simulink model "Filtri_Statici"  (R2022b)
settings: Solver=VariableStepAuto  StartTime=0.0  StopTime=time_max  FixedStep=1e-6  RelTol=1e-4
values from neighbouring files (symbols this model uses):
  bias_accel = [bias_a_x; bias_a_y; bias_a_z]    [Main_Articolo.m]
  bias_csi = [bias_csi_x; bias_csi_y; bias_csi_z]    [Main_Articolo.m]
  bias_gyro = [bias_gyro_x; bias_gyro_y; bias_gyro_z]    [Main_Articolo.m]    (also in Plot_Filtri_Din.m = out.bias_gyro.Data)
  bias_magn = [bias_magn_x; bias_magn_y; bias_magn_z]    [Main_Articolo.m]
  csi_i = [0; csi_y_i; 0]    [Main_Articolo.m]
  dev_std_a_x = 0.0248    [Main_Articolo.m]
  dev_std_a_y = 0.0248    [Main_Articolo.m]
  dev_std_a_z = 0.0203    [Main_Articolo.m]
  dev_std_csi_x = 0.01    [Main_Articolo.m]
  dev_std_csi_y = 0.007    [Main_Articolo.m]
  dev_std_csi_z = 0.005    [Main_Articolo.m]
  dev_std_gyro_x = 2.653*10^(-3)    (= 0.002653)    [Main_Articolo.m]
  dev_std_gyro_y = 2.653*10^(-3)    (= 0.002653)    [Main_Articolo.m]
  dev_std_gyro_z = 3.159*10^(-3)    (= 0.003159)    [Main_Articolo.m]
  dev_std_magn_x = 0.01    [Main_Articolo.m]
  dev_std_magn_y = 0.015    [Main_Articolo.m]
  dev_std_magn_z = 0.0175    [Main_Articolo.m]
  dt = 0.01    [Main_Articolo.m]
  flag = 1    [Main_Articolo.m]
  g = 9.81    [Main_Articolo.m]
  index = 0    [Main_Articolo.m]
  k_accel = 1/3    (= 0.333333333333)    [Main_Articolo.m]
  k_csi = 1/3    (= 0.333333333333)    [Main_Articolo.m]
  k_magn = 1/3    (= 0.333333333333)    [Main_Articolo.m]
  m_I = [m_i_x; 0; m_i_z]    [Main_Articolo.m]
  Omega11 = 0.075    [Main_Articolo.m]
  Omega12 = 0.045    [Main_Articolo.m]
  Omega13 = 0.02    [Main_Articolo.m]
  Omega21 = 0.085    [Main_Articolo.m]
  Omega22 = -0.03    [Main_Articolo.m]
  Omega23 = 0.015    [Main_Articolo.m]
  Omega31 = 0.1    [Main_Articolo.m]
  Omega32 = 0.036    [Main_Articolo.m]
  Omega33 = -0.025    [Main_Articolo.m]
  Phi1 = 40*pi/180    (= 0.698131700798)    [Main_Articolo.m]
  Phi2 = 20*pi/180    (= 0.349065850399)    [Main_Articolo.m]
  Phi3 = 2*pi/180    (= 0.0349065850399)    [Main_Articolo.m]
  phi_0 = 15*pi/180    (= 0.261799387799)    [Main_Articolo.m]
  pos_0 = [x_0; y_0; z_0]    [Main_Articolo.m]
  Psi1 = 160*pi/180    (= 2.79252680319)    [Main_Articolo.m]
  Psi2 = 35*pi/180    (= 0.610865238198)    [Main_Articolo.m]
  Psi3 = 5*pi/180    (= 0.0872664625997)    [Main_Articolo.m]
  psi_0 = pi/4    (= 0.785398163397)    [Main_Articolo.m]
  rumori_bias = 1    [Main_Articolo.m]
  Theta1 = 50*pi/180    (= 0.872664625997)    [Main_Articolo.m]
  Theta2 = 12*pi/180    (= 0.209439510239)    [Main_Articolo.m]
  Theta3 = 3*pi/180    (= 0.0523598775598)    [Main_Articolo.m]
  theta_0 = 10*pi/180    (= 0.174532925199)    [Main_Articolo.m]
  Ttriad = 1/30    (= 0.0333333333333)    [Main_Articolo.m]
  vel_0 = [dx_0; dy_0; dz_0]    [Main_Articolo.m]
  w_11 = 2*pi/30    (= 0.209439510239)    [Main_Articolo.m]
  w_12 = 2*pi/12    (= 0.523598775598)    [Main_Articolo.m]
  w_13 = 2*pi/4    (= 1.57079632679)    [Main_Articolo.m]
  w_21 = 2*pi/25    (= 0.251327412287)    [Main_Articolo.m]
  w_22 = 2*pi/18    (= 0.349065850399)    [Main_Articolo.m]
  w_23 = 2*pi/3    (= 2.09439510239)    [Main_Articolo.m]
  w_31 = 2*pi/20    (= 0.314159265359)    [Main_Articolo.m]
  w_32 = 2*pi/10    (= 0.628318530718)    [Main_Articolo.m]
  w_33 = 2*pi/2    (= 3.14159265359)    [Main_Articolo.m]
  w_phi1 = 2*pi/27    (= 0.232710566933)    [Main_Articolo.m]
  w_phi2 = 2*pi/18    (= 0.349065850399)    [Main_Articolo.m]
  w_phi3 = 2*pi/3    (= 2.09439510239)    [Main_Articolo.m]
  w_psi1 = 2*pi/30    (= 0.209439510239)    [Main_Articolo.m]
  w_psi2 = 2*pi/15    (= 0.418879020479)    [Main_Articolo.m]
  w_psi3 = 2*pi/4    (= 1.57079632679)    [Main_Articolo.m]
  w_theta1 = 2*pi/23    (= 0.273181969877)    [Main_Articolo.m]
  w_theta2 = 2*pi/12    (= 0.523598775598)    [Main_Articolo.m]
  w_theta3 = 2*pi/3.5    (= 1.79519580205)    [Main_Articolo.m]
settings Model: Creator=paoga  LastModifiedBy=paoga

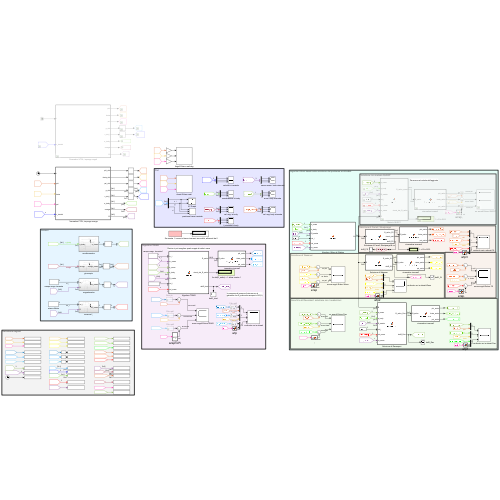
[thumbnail: Simulink's stored preview of the top-level diagram]
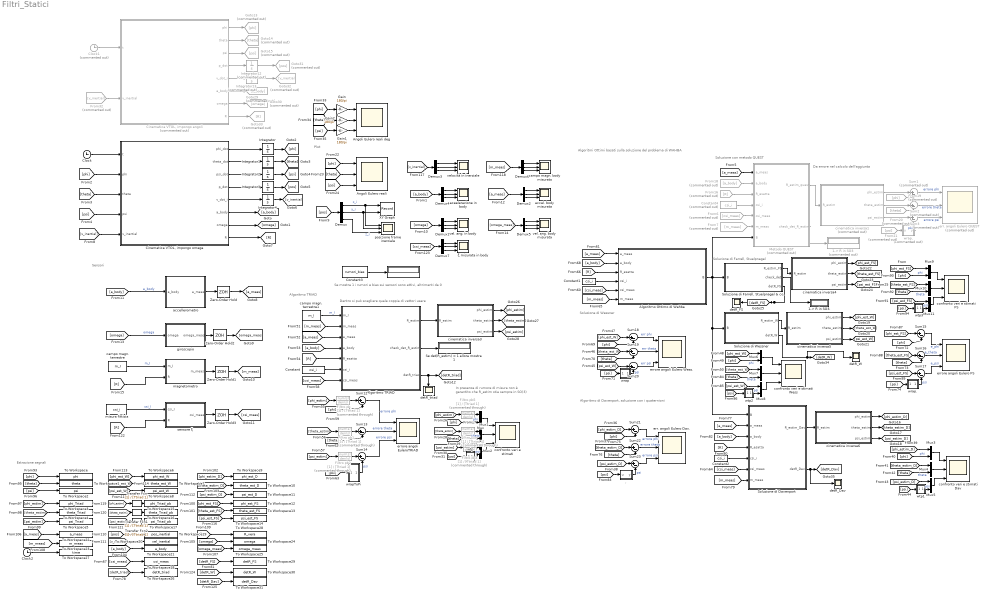
== system Filtri_Statici ==
  note: Da errore nel calcolo dell'aggiunta
  note: Algoritmi Ottimi basati sulla soluzione del problema di WAHBA
  note: Soluzione con metodo QUEST
  note: Algoritmo di Davenport, soluzione con i quaternioni
  note: Plot
  note: Sensori
  note: Dentro si può scegliere quale coppia di vettori usare
  note: In presenza di rumore di misura non è
      | garantito che R_estim stia sempre in SO(3)
  note: Algoritmo TRIAD
  note: Soluzione di Wessner
  note: Soluzione di Farrell, Stuelpnagel
  note: Se mostra 1 i rumori e bias sui sensori sono attivi, altrimenti da 0
  note: Estrazione segnali
  , : MATLAB Function  TreatAsAtomicUnit=on
  . : Display
  1-> R in SO3 : Display  Commented=on
  1-> R in SO3. : Display
  Algoritmo Ottimo di Wahba : MATLAB Function  TreatAsAtomicUnit=on
  Algoritmo TRIAD : MATLAB Function  TreatAsAtomicUnit=on
  Angoli Eulero reali : Scope  NumInputPorts=3
  Angoli Eulero reali deg : Scope  NumInputPorts=3
  "Cinematica VTOL, impongo angoli" : MATLAB Function  Commented=on  TreatAsAtomicUnit=on
  "Cinematica VTOL, impongo omega" : MATLAB Function  TreatAsAtomicUnit=on
  Clock : Clock
  Clock1 : Clock  Commented=on
  Clock2 : Clock
  Constant : Constant  Value=csi_i
  Constant1 : Constant  Value=csi_i
  Constant2 : Constant  Value=csi_i
  Constant3 : Constant  Value=rumori_bias
  Constant4 : Constant  Commented=on  Value=csi_i
  Demux{,1..7} (8 alike) : Demux  Outputs=3
  Filtro pb{,1..5} (6 alike) : TransferFcn  Commented=through  Denominator=[Ttriad 1]
  From16 : From  Commented=on  GotoTag=R
  From18 : From  Commented=on  GotoTag=a_body
  From19 : From  Commented=on  GotoTag=phi
  From20 : From  Commented=on  GotoTag=theta
  From21 : From  Commented=on  GotoTag=psi
  From32 : From  Commented=on  GotoTag=v_inertial
  From6 : From  Commented=on  GotoTag=csi_meas
  From7 : From  Commented=on  GotoTag=m_meas
  Gain : Gain  Gain=180/pi
  Gain1 : Gain  Gain=180/pi
  Gain2 : Gain  Gain=180/pi
  Goto13 : Goto  Commented=on  GotoTag=phi
  Goto14 : Goto  Commented=on  GotoTag=theta
  Goto15 : Goto  Commented=on  GotoTag=psi
  Goto29 : Goto  Commented=on  GotoTag=a_body
  Goto30 : Goto  Commented=on  GotoTag=omega
  Goto31 : Goto  Commented=on  GotoTag=pos
  Goto32 : Goto  Commented=on  GotoTag=v_inertial
  Goto33 : Goto  Commented=on  GotoTag=R
  Integrator : Integrator  InitialCondition=phi_0
  Integrator1 : Integrator  InitialCondition=theta_0
  Integrator12 : Integrator  Commented=on  InitialCondition=pos_0
  Integrator13 : Integrator  Commented=on  InitialCondition=vel_0
  Integrator2 : Integrator  InitialCondition=psi_0
  Integrator3 : Integrator  InitialCondition=pos_0
  Integrator4 : Integrator  InitialCondition=vel_0
  Metodo QUEST : MATLAB Function  Commented=on  TreatAsAtomicUnit=on
  Mux{,1..11} (12 alike) : Mux  Inputs=2
  Se det(R_estim) = 1 allora mostra 1 : Display
  Soluzione di Davenport : MATLAB Function  TreatAsAtomicUnit=on
  "Soluzione di Farrell, Stuelpnagel & co." : MATLAB Function  TreatAsAtomicUnit=on
  Soluzione di Wessner : MATLAB Function  TreatAsAtomicUnit=on
  Sum1 : Sum  Commented=on  Inputs=|+-
  Sum{12..23} (12 alike) : Sum  Inputs=|+-
  Sum2 : Sum  Commented=on  Inputs=|+-
  Sum3 : Sum  Commented=on  Inputs=|+-
  To Workspace : ToWorkspace  VariableName=phi  SaveFormat=Timeseries  SampleTime=-1
  To Workspace1 : ToWorkspace  VariableName=theta  SaveFormat=Timeseries  SampleTime=-1
  To Workspace10 : ToWorkspace  VariableName=theta_est_D  SaveFormat=Timeseries  SampleTime=-1
  To Workspace11 : ToWorkspace  VariableName=psi_est_D  SaveFormat=Timeseries  SampleTime=-1
  To Workspace12 : ToWorkspace  VariableName=phi_est_FS  SaveFormat=Timeseries  SampleTime=-1
  To Workspace13 : ToWorkspace  VariableName=theta_est_FS  SaveFormat=Timeseries  SampleTime=-1
  To Workspace14 : ToWorkspace  VariableName=psi_est_FS  SaveFormat=Timeseries  SampleTime=-1
  To Workspace15 : ToWorkspace  VariableName=phi_Triad_pb  SaveFormat=Timeseries  SampleTime=-1
  To Workspace16 : ToWorkspace  VariableName=theta_Triad_pb  SaveFormat=Timeseries  SampleTime=-1
  To Workspace17 : ToWorkspace  VariableName=psi_Triad_pb  SaveFormat=Timeseries  SampleTime=-1
  To Workspace18 : ToWorkspace  VariableName=csi_meas  SaveFormat=Timeseries  SampleTime=-1
  To Workspace19 : ToWorkspace  VariableName=pos_inertial  SaveFormat=Timeseries  SampleTime=-1
  To Workspace2 : ToWorkspace  VariableName=psi  SaveFormat=Timeseries  SampleTime=-1
  To Workspace20 : ToWorkspace  VariableName=vel_inertial  SaveFormat=Timeseries  SampleTime=-1
  To Workspace21 : ToWorkspace  VariableName=a_body  SaveFormat=Timeseries  SampleTime=-1
  To Workspace22 : ToWorkspace  VariableName=a_meas  SaveFormat=Timeseries  SampleTime=-1
  To Workspace23 : ToWorkspace  VariableName=m_meas  SaveFormat=Timeseries  SampleTime=-1
  To Workspace24 : ToWorkspace  VariableName=omega  SaveFormat=Timeseries  SampleTime=-1
  To Workspace25 : ToWorkspace  VariableName=omega_meas  SaveFormat=Timeseries  SampleTime=-1
  To Workspace26 : ToWorkspace  VariableName=detR_triad  SaveFormat=Timeseries  SampleTime=-1
  To Workspace27 : ToWorkspace  VariableName=time  SampleTime=-1
  To Workspace28 : ToWorkspace  VariableName=R_vera  SampleTime=-1
  To Workspace29 : ToWorkspace  VariableName=detR_FS  SaveFormat=Timeseries  SampleTime=-1
  To Workspace3 : ToWorkspace  VariableName=phi_Triad  SaveFormat=Timeseries  SampleTime=-1
  To Workspace30 : ToWorkspace  VariableName=detR_W  SaveFormat=Timeseries  SampleTime=-1
  To Workspace31 : ToWorkspace  VariableName=detR_Dav  SaveFormat=Timeseries  SampleTime=-1
  To Workspace4 : ToWorkspace  VariableName=theta_Triad  SaveFormat=Timeseries  SampleTime=-1
  To Workspace5 : ToWorkspace  VariableName=psi_Triad  SaveFormat=Timeseries  SampleTime=-1
  To Workspace6 : ToWorkspace  VariableName=phi_est_W  SaveFormat=Timeseries  SampleTime=-1
  To Workspace7 : ToWorkspace  VariableName=theta_est_W  SaveFormat=Timeseries  SampleTime=-1
  To Workspace8 : ToWorkspace  VariableName=psi_est_W  SaveFormat=Timeseries  SampleTime=-1
  To Workspace9 : ToWorkspace  VariableName=phi_est_D  SaveFormat=Timeseries  SampleTime=-1
  Transfer Fcn : TransferFcn  Denominator=[Ttriad 1]
  Transfer Fcn1 : TransferFcn  Denominator=[Ttriad 1]
  Transfer Fcn2 : TransferFcn  Denominator=[Ttriad 1]
  XY Graph : Record  FileSettingsInternal="{\"entries\":[{\"content\":{\"excelSettings\":{\"content\":{},\"type\":\"Streamout.ExcelSettings\"}},\"type\":\"Streamout.FileSettingStorage\",\"uuid\":\"477e70b2-955e-4b5a-84c2-a5f2bc9940fe\"}],\"packageUris\":[\"http://schema.mathworks.com/mf0/streamout_blocks/R2020a\"],\"version\":\"1.0\"}"  Layout=[1 1]  SignalsInternal="{\"entries\":[{\"content\":{\"signals\":[{\"content\":{\"blockPath\":[\"Filtri_Statici/XY Graph\"],\"channel\":[],\"dimensions\":[1,1],\"domain\":\"Filtri_Statici/XY Graph\",\"lineColor\":\"#a2142f\",\"plots\":[1],\"port\":1,\"sid\":[\"\"],\"signalID\":3592,\"signalName\":\"x_i\"},\"type\":\"RecordBlkView.Signal\",\"uuid\":\"d6606014-7fdd-4c5b-a990-e5a37003c0d6\"},{\"content\":{\"blockPath\":[\"Filtri_Statici/XY Graph\"],\"channel\":[],\"dimensions\":[1,1],\"domain\":\"Filtri_Statici/XY Graph\",\"lineColor\":\"#139fff\",\"plots\":[1],\"port\":2,\"sid\":[\"\"],\"signalID\":3596,\"signalName\":\"y_i\"},\"type\":\"RecordBlkView.Signal\",\"uuid\":\"6f7c022e-9ea7-4631-a991-0923b55dc0a6\"}]},\"type\":\"RecordBlkView.InputSignals\",\"uuid\":\"fece2fe3-a12d-44ca-a4d1-88af198f26aa\"}],\"packageUris\":[\"http://schema.mathworks.com/mf0/streamout_blocks/R2020a\"],\"version\":\"1.0\"}"  VisualizationBindings="{\"xyplotplugin\":{\"info\":[{\"series\":[{\"bindingParametersList\":[{\"parameter\":\"X-Axis\",\"signalID\":3592,\"signalName\":\"x_i\"},{\"parameter\":\"Y-Axis\",\"signalID\":3596,\"signalName\":\"y_i\"}],\"seriesID\":16300}],\"subplotID\":1}]}}"  CompatibilityTag=XY
  Zero-Order Hold{,1..3} (4 alike) : ZeroOrderHold  SampleTime=dt
  accel. body misurata : Scope  NumInputPorts=3
  accellerometro : Subsystem
  aceelerazione in body : Scope  NumInputPorts=3
  campo magn. body misurato : Scope  NumInputPorts=3
  campo magn. terrestre : Constant  Value=m_I
  campo magn. terrestre1 : Constant  Value=m_I
  cinematica inversa1 : MATLAB Function  Commented=on  TreatAsAtomicUnit=on
  cinematica inversa3 : MATLAB Function  TreatAsAtomicUnit=on
  cinematica inversa4 : MATLAB Function  TreatAsAtomicUnit=on
  cinematica inversa5 : MATLAB Function  TreatAsAtomicUnit=on
  cinematica inversa6 : MATLAB Function  TreatAsAtomicUnit=on
  confronto veri e stimati : Scope  NumInputPorts=3
  confronto veri e stimati Dav : Scope  NumInputPorts=3
  confronto veri e stimati FS : Scope  NumInputPorts=3
  confronto veri e stimati Wess : Scope  NumInputPorts=3
  detR_Dav : Scope
  detR_FS : Scope
  detR_W : Scope
  detR_triad : Scope
  err. angoli Eulero Dav. : Scope  NumInputPorts=3
  err. angoli Eulero QUEST : Scope  Commented=on  NumInputPorts=3
  errore angoli Eulero FS : Scope  NumInputPorts=3
  errore angoli Eulero Wess. : Scope  NumInputPorts=3
  errore angoli EuleroTRIAD : Scope  NumInputPorts=3
  giroscopio : Subsystem
  magnetometro : Subsystem
  misura fittizia : Constant  Value=csi_i
  posizione frame inerziale : Scope  NumInputPorts=3
  "sensore ξ " : Subsystem
  vel. ang. body misurata : Scope  NumInputPorts=3
  vel. ang. in body : Scope  NumInputPorts=3
  velocità in inerziale : Scope  NumInputPorts=3
  wrap : MATLAB Function  TreatAsAtomicUnit=on
  wrap, : MATLAB Function  Commented=on  TreatAsAtomicUnit=on
  wrap. : MATLAB Function  TreatAsAtomicUnit=on
  wrapToPi : MATLAB Function  TreatAsAtomicUnit=on
  wtp : MATLAB Function  TreatAsAtomicUnit=on
  wtp1 : MATLAB Function  TreatAsAtomicUnit=on
  wtp2 : MATLAB Function  TreatAsAtomicUnit=on
  wtp3 : MATLAB Function  TreatAsAtomicUnit=on
  ξ misurata in body : Scope  NumInputPorts=3
  wires:
  Demux1/3 -> vel. ang. in body/3
  "Cinematica VTOL, impongo omega"/6(a_body) -> [a_body]
  Integrator/1 -> [phi]
  [psi] -> "Cinematica VTOL, impongo omega"/4(psi)
  [omega] -> Demux1/1
  Clock/1 -> "Cinematica VTOL, impongo omega"/1(t)
  Demux5/3 -> vel. ang. body misurata/3
  Integrator4/1 -> [v_inertial]
  Demux4/1 -> aceelerazione in body/1
  Integrator2/1 -> [psi]
  Constant3/1 -> ./1
  [a_meas] -> Demux2/1
  [omega_meas] -> Demux5/1
  [a_body] -> Demux4/1
  Demux4/2 -> aceelerazione in body/2
  "Cinematica VTOL, impongo omega"/7(omega) -> [omega]
  [pos] -> Demux/1
  Demux/1 -> posizione frame inerziale/1, XY Graph/1  "x_i"
  [phi] -> "Cinematica VTOL, impongo omega"/2(phi)
  Integrator3/1 -> [pos]
  Demux2/1 -> accel. body misurata/1
  Demux2/2 -> accel. body misurata/2
  [v_inertial] -> "Cinematica VTOL, impongo omega"/5(v_inertial)
  Demux5/2 -> vel. ang. body misurata/2
  Demux4/3 -> aceelerazione in body/3
  "Cinematica VTOL, impongo omega"/4(p_dot) -> Integrator3/1
  Demux/3 -> posizione frame inerziale/3  "z_i"
  Demux2/3 -> accel. body misurata/3
  Demux1/1 -> vel. ang. in body/1
  Demux1/2 -> vel. ang. in body/2
  "Cinematica VTOL, impongo omega"/3(psi_dot) -> Integrator2/1
  "Cinematica VTOL, impongo omega"/2(theta_dot) -> Integrator1/1
  Demux5/1 -> vel. ang. body misurata/1
  "Cinematica VTOL, impongo omega"/8(R) -> [R]
  Integrator1/1 -> [theta]
  "Cinematica VTOL, impongo omega"/1(phi_dot) -> Integrator/1
  Demux/2 -> posizione frame inerziale/2, XY Graph/2  "y_i"
  [theta] -> "Cinematica VTOL, impongo omega"/3(theta)
  "Cinematica VTOL, impongo omega"/5(v_dot_i) -> Integrator4/1
  accellerometro/1(a_meas) -> Zero-Order Hold/1
  [a_body] -> accellerometro/1(a_body)  "a_body"
  Zero-Order Hold2/1 -> [omega_meas]
  giroscopio/1(omega_meas) -> Zero-Order Hold2/1
  Zero-Order Hold1/1 -> [m_meas]
  [omega] -> giroscopio/1(omega)  "omega"
  [R] -> magnetometro/2(R)
  Zero-Order Hold/1 -> [a_meas]
  magnetometro/1(m_meas) -> Zero-Order Hold1/1
  campo magn. terrestre/1 -> magnetometro/1(m_I)  "m_I"
  Sum14/1 -> errore angoli EuleroTRIAD/3  "errore psi"
  Sum12/1 -> errore angoli EuleroTRIAD/1  "errore phi"
  [psi_estim] -> Filtro pb2/1
  Algoritmo TRIAD/1(R_estim) -> cinematica inversa3/1(R_estim)
  [a_meas] -> Algoritmo TRIAD/3(a_meas)
  Algoritmo TRIAD/3(detR_triad) -> [detR_triad], detR_triad/1
  [a_body] -> Algoritmo TRIAD/4(a_body)
  [psi] -> wrapToPi/1(u)
  campo magn. terrestre1/1 -> Algoritmo TRIAD/1(m_I)  "m_I"
  [theta] -> Sum13/2
  cinematica inversa3/1(phi_estim) -> [phi_estim]
  cinematica inversa3/2(theta_estim) -> [theta_estim]
  Constant/1 -> Algoritmo TRIAD/6(csi_i)
  Algoritmo TRIAD/2(check_det_R_estim) -> Se det(R_estim) = 1 allora mostra 1/1
  [csi_meas] -> Algoritmo TRIAD/7(csi_meas)
  [phi_estim] -> Filtro pb/1
  cinematica inversa3/3(psi_estim) -> [psi_estim]
  [phi] -> Sum12/2
  [R] -> Algoritmo TRIAD/5(R_esatta)
  [m_meas] -> Algoritmo TRIAD/2(m_meas)
  [theta_estim] -> Filtro pb1/1
  Sum13/1 -> errore angoli EuleroTRIAD/2  "errore theta"
  cinematica inversa6/2(theta_estim) -> [theta_estim_D]
  [m_meas] -> Soluzione di Davenport/7(m_meas)
  Soluzione di Davenport/1(R_estim_Dav) -> cinematica inversa6/1(R_estim)
  Sum16/1 -> errore angoli Eulero FS/2  "e_theta"
  Sum21/1 -> err. angoli Eulero Dav./1  "errore phi"
  [R] -> Algoritmo Ottimo di Wahba/3(R_esatta)
  [psi] -> ,/1(u)
  [m_meas] -> Algoritmo Ottimo di Wahba/6(m_meas)
  cinematica inversa5/1(phi_estim) -> [phi_est_W]
  [csi_meas] -> Soluzione di Davenport/6(csi_meas)
  Constant2/1 -> Soluzione di Davenport/5(csi_i)
  cinematica inversa4/1(phi_estim) -> [phi_est_FS]
  [phi] -> Sum15/2
  Sum22/1 -> err. angoli Eulero Dav./2  "errore theta"
  [theta] -> Sum22/2
  Sum23/1 -> err. angoli Eulero Dav./3  "errore psi"
  [a_body] -> Algoritmo Ottimo di Wahba/2(a_body)
  cinematica inversa6/3(psi_estim) -> [psi_estim_D]
  [csi_meas] -> Algoritmo Ottimo di Wahba/5(csi_meas)
  Sum17/1 -> errore angoli Eulero FS/3  "e_psi"
  "Soluzione di Farrell, Stuelpnagel & co."/1(R_estim_FS) -> cinematica inversa4/1(R_estim)
  Soluzione di Wessner/1(R_estim_W) -> cinematica inversa5/1(R_estim)
  [psi] -> wrap./1(u)
  [psi] -> wrap/1(u)
  cinematica inversa6/1(phi_estim) -> [phi_estim_D]
  cinematica inversa4/2(theta_estim) -> [theta_est_FS]
  cinematica inversa4/3(psi_estim) -> [psi_est_FS]
  [theta] -> Sum16/2
  Constant1/1 -> Algoritmo Ottimo di Wahba/4(csi_i)
  Sum19/1 -> errore angoli Eulero Wess./2  "err theta"
  Algoritmo Ottimo di Wahba/1(B) -> Soluzione di Davenport/1(B), Soluzione di Wessner/1(B), "Soluzione di Farrell, Stuelpnagel & co."/1(B), Metodo QUEST/7(B)
  [theta] -> Sum19/2
  cinematica inversa5/3(psi_estim) -> [psi_est_W]
  [phi] -> Sum18/2
  [phi] -> Sum21/2
  cinematica inversa5/2(theta_estim) -> [theta_est_W]
  Sum18/1 -> errore angoli Eulero Wess./1  "err phi"
  [R] -> Soluzione di Davenport/4(R_esatta)
  Sum15/1 -> errore angoli Eulero FS/1  "e_phi"
  [a_meas] -> Algoritmo Ottimo di Wahba/1(a_meas)
  [a_body] -> Soluzione di Davenport/3(a_body)
  [a_meas] -> Soluzione di Davenport/2(a_meas)
  Sum20/1 -> errore angoli Eulero Wess./3  "err psi"
  From6/1 -> Metodo QUEST/5(csi_meas)
  [a_meas] -> Metodo QUEST/1(a_meas)
  From18/1 -> Metodo QUEST/2(a_body)
  From16/1 -> Metodo QUEST/3(R_esatta)
  Constant4/1 -> Metodo QUEST/4(csi_i)
  From7/1 -> Metodo QUEST/6(m_meas)
  From20/1 -> Sum2/2
  From19/1 -> Sum1/2
  Sum2/1 -> err. angoli Eulero QUEST/2  "errore theta"
  Sum3/1 -> err. angoli Eulero QUEST/3  "errore psi"
  Sum1/1 -> err. angoli Eulero QUEST/1  "errore phi"
  From21/1 -> wrap,/1(u)
  Metodo QUEST/1(R_estim_quest) -> cinematica inversa1/1(R_estim)
  cinematica inversa1/1(phi_estim) -> Sum1/1
  cinematica inversa1/2(theta_estim) -> Sum2/1
  cinematica inversa1/3(psi_estim) -> Sum3/1
  [phi] -> Angoli Eulero reali/1
  [psi] -> Angoli Eulero reali/3
  [theta] -> Angoli Eulero reali/2
  Metodo QUEST/2(check_det_R_estim) -> 1-> R in SO3/1
  "Soluzione di Farrell, Stuelpnagel & co."/2(check_det) -> 1-> R in SO3./1
  Soluzione di Davenport/2(detR_Dav) -> detR_Dav/1, [detR_Dav]
  wrapToPi/1(y) -> Sum14/2  "psi"
  ,/1(y) -> Sum23/2  "psi"
  wrap/1(y) -> Sum20/2  "psi"
  wrap./1(y) -> Sum17/2  "psi"
  wrap,/1(y) -> Sum3/2  "psi"
  Mux1/1 -> confronto veri e stimati/2
  Mux/1 -> confronto veri e stimati/1
  [theta] -> Mux1/2  "theta"
  [phi] -> Mux/2  "phi"
  Mux2/1 -> confronto veri e stimati/3
  [theta_estim] -> Filtro pb4/1
  [psi] -> wtp/1(u)
  wtp/1(y) -> Mux2/2  "psi"
  [phi_estim] -> Filtro pb5/1
  "Cinematica VTOL, impongo angoli"/6(a_body) -> Goto29/1
  Integrator13/1 -> Goto32/1
  "Cinematica VTOL, impongo angoli"/2(theta) -> Goto14/1
  From32/1 -> "Cinematica VTOL, impongo angoli"/2(v_inertial)
  "Cinematica VTOL, impongo angoli"/4(p_dot) -> Integrator12/1
  "Cinematica VTOL, impongo angoli"/5(v_dot_i) -> Integrator13/1
  Integrator12/1 -> Goto31/1
  "Cinematica VTOL, impongo angoli"/7(omega) -> Goto30/1
  "Cinematica VTOL, impongo angoli"/3(psi) -> Goto15/1
  Clock1/1 -> "Cinematica VTOL, impongo angoli"/1(t)
  "Cinematica VTOL, impongo angoli"/8(R) -> Goto33/1
  "Cinematica VTOL, impongo angoli"/1(phi) -> Goto13/1
  Gain1/1 -> Angoli Eulero reali deg/3
  [psi] -> Gain1/1
  Gain/1 -> Angoli Eulero reali deg/1
  Gain2/1 -> Angoli Eulero reali deg/2
  [phi] -> Gain/1
  [theta] -> Gain2/1
  [phi_estim_D] -> Sum21/1
  [theta_estim_D] -> Sum22/1
  [psi_estim_D] -> Sum23/1
  [psi_estim_D] -> Mux5/1
  [theta] -> Mux4/2  "theta"
  [theta_estim_D] -> Mux4/1
  [psi] -> wtp1/1(u)
  [phi_estim_D] -> Mux3/1
  wtp1/1(y) -> Mux5/2  "psi"
  Mux5/1 -> confronto veri e stimati Dav/3
  Mux3/1 -> confronto veri e stimati Dav/1
  [phi] -> Mux3/2  "phi"
  Mux4/1 -> confronto veri e stimati Dav/2
  [psi_est_W] -> Sum20/1
  [theta_est_W] -> Sum19/1
  [phi_est_W] -> Sum18/1
  [theta_est_W] -> Mux7/1
  [phi] -> Mux6/2  "phi"
  Mux8/1 -> confronto veri e stimati Wess/3
  wtp2/1(y) -> Mux8/2  "psi"
  [psi] -> wtp2/1(u)
  [theta] -> Mux7/2  "theta"
  [psi_est_W] -> Mux8/1
  Mux6/1 -> confronto veri e stimati Wess/1
  Mux7/1 -> confronto veri e stimati Wess/2
  [phi_est_FS] -> Sum15/1
  [theta_est_FS] -> Sum16/1
  [psi_est_FS] -> Sum17/1
  [theta_est_FS] -> Mux10/1
  [phi] -> Mux9/2  "phi"
  Mux11/1 -> confronto veri e stimati FS/3
  wtp3/1(y) -> Mux11/2  "psi"
  [psi] -> wtp3/1(u)
  [theta] -> Mux10/2  "theta"
  [psi_est_FS] -> Mux11/1
  Mux9/1 -> confronto veri e stimati FS/1
  Mux10/1 -> confronto veri e stimati FS/2
  Clock2/1 -> To Workspace27/1
  [v_inertial] -> To Workspace20/1
  [phi_est_FS] -> To Workspace12/1
  [phi_est_W] -> To Workspace6/1
  [m_meas] -> To Workspace23/1
  [pos] -> To Workspace19/1
  [psi_est_W] -> To Workspace8/1
  [theta_est_FS] -> To Workspace13/1
  [theta_est_W] -> To Workspace7/1
  [psi] -> To Workspace2/1
  [psi_estim_D] -> To Workspace11/1
  [a_body] -> To Workspace21/1
  [a_meas] -> To Workspace22/1
  [theta_estim] -> To Workspace4/1
  [psi_estim] -> To Workspace5/1
  [psi_est_FS] -> To Workspace14/1
  [theta] -> To Workspace1/1
  [phi_estim_D] -> To Workspace9/1
  [phi_estim] -> To Workspace3/1
  [theta_estim_D] -> To Workspace10/1
  [omega] -> To Workspace24/1
  [phi] -> To Workspace/1
  [omega_meas] -> To Workspace25/1
  [R] -> To Workspace28/1
  Filtro pb/1 -> Sum12/1
  Filtro pb1/1 -> Sum13/1
  Filtro pb2/1 -> Sum14/1
  Filtro pb5/1 -> Mux/1
  Filtro pb4/1 -> Mux1/1
  [psi_estim] -> Filtro pb3/1
  Filtro pb3/1 -> Mux2/1
  Demux6/2 -> campo magn. body misurato/2
  Demux3/3 -> velocità in inerziale/3
  Demux3/1 -> velocità in inerziale/1
  [m_meas] -> Demux6/1
  [v_inertial] -> Demux3/1
  Demux6/1 -> campo magn. body misurato/1
  Demux3/2 -> velocità in inerziale/2
  Demux6/3 -> campo magn. body misurato/3
  [phi_estim] -> Transfer Fcn/1
  Transfer Fcn/1 -> To Workspace15/1
  [theta_estim] -> Transfer Fcn1/1
  Transfer Fcn1/1 -> To Workspace16/1
  [psi_estim] -> Transfer Fcn2/1
  Transfer Fcn2/1 -> To Workspace17/1
  [phi_est_FS] -> Mux9/1
  [phi_est_W] -> Mux6/1
  [R] -> "sensore ξ "/2(R)
  misura fittizia/1 -> "sensore ξ "/1(csi_I)  "csi_I"
  Zero-Order Hold3/1 -> [csi_meas]
  "sensore ξ "/1(csi_meas) -> Zero-Order Hold3/1
  Demux7/3 -> ξ misurata in body/3
  Demux7/2 -> ξ misurata in body/2
  [csi_meas] -> Demux7/1
  Demux7/1 -> ξ misurata in body/1
  [csi_meas] -> To Workspace18/1
  [detR_triad] -> To Workspace26/1
  "Soluzione di Farrell, Stuelpnagel & co."/3(detR_FS) -> detR_FS/1, [detR_FS]
  [detR_FS] -> To Workspace29/1
  Soluzione di Wessner/2(detR_W) -> detR_W/1, [detR_W]
  [detR_W] -> To Workspace30/1
  [detR_Dav] -> To Workspace31/1

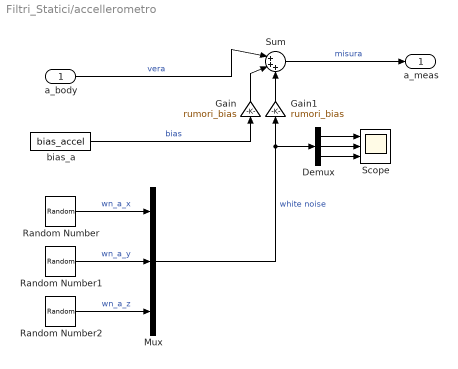
== system Filtri_Statici/accellerometro ==
  a_body : Inport
  Demux : Demux  Outputs=3
  Gain : Gain  Gain=rumori_bias
  Gain1 : Gain  Gain=rumori_bias
  Mux : Mux  Inputs=3
  Random Number : RandomNumber  Variance=dev_std_a_x^2  Seed=1  SampleTime=dt
  Random Number1 : RandomNumber  Variance=dev_std_a_y^2  Seed=2  SampleTime=dt
  Random Number2 : RandomNumber  Variance=dev_std_a_z^2  Seed=3  SampleTime=dt
  Scope : Scope  NumInputPorts=3
  Sum : Sum  Inputs=|+++
  bias_a : Constant  Value=bias_accel
  a_meas : Outport
  wires:
  Random Number2/1 -> Mux/3  "wn_a_z"
  bias_a/1 -> Gain/1  "bias"
  Sum/1 -> a_meas/1  "misura"
  a_body/1 -> Sum/1  "vera"
  Random Number1/1 -> Mux/2  "wn_a_y"
  Mux/1 -> Demux/1, Gain1/1  "white noise"
  Random Number/1 -> Mux/1  "wn_a_x"
  Demux/1 -> Scope/1
  Demux/2 -> Scope/2
  Demux/3 -> Scope/3
  Gain/1 -> Sum/2
  Gain1/1 -> Sum/3

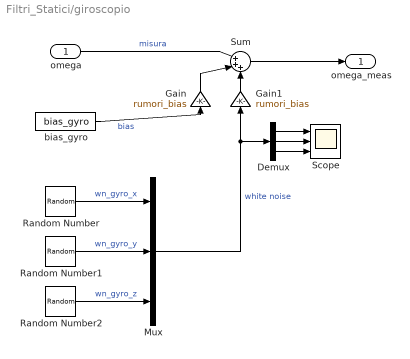
== system Filtri_Statici/giroscopio ==
  omega : Inport
  Demux : Demux  Outputs=3
  Gain : Gain  Gain=rumori_bias
  Gain1 : Gain  Gain=rumori_bias
  Mux : Mux  Inputs=3
  Random Number : RandomNumber  Variance=dev_std_gyro_x^2  Seed=4  SampleTime=dt
  Random Number1 : RandomNumber  Variance=dev_std_gyro_y^2  Seed=5  SampleTime=dt
  Random Number2 : RandomNumber  Variance=dev_std_gyro_z^2  Seed=6  SampleTime=dt
  Scope : Scope  NumInputPorts=3
  Sum : Sum  Inputs=|+++
  bias_gyro : Constant  Value=bias_gyro
  omega_meas : Outport
  wires:
  Sum/1 -> omega_meas/1
  omega/1 -> Sum/1  "misura"
  Demux/2 -> Scope/2
  Demux/3 -> Scope/3
  Mux/1 -> Demux/1, Gain1/1  "white noise"
  Demux/1 -> Scope/1
  Random Number2/1 -> Mux/3  "wn_gyro_z"
  Random Number/1 -> Mux/1  "wn_gyro_x"
  Random Number1/1 -> Mux/2  "wn_gyro_y"
  bias_gyro/1 -> Gain/1  "bias"
  Gain1/1 -> Sum/3
  Gain/1 -> Sum/2

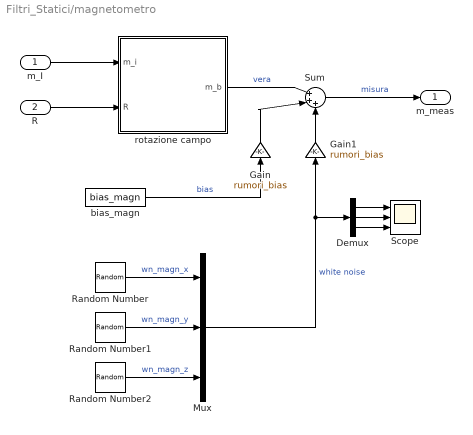
== system Filtri_Statici/magnetometro ==
  m_I : Inport
  R : Inport  Port=2
  Demux : Demux  Outputs=3
  Gain : Gain  Gain=rumori_bias
  Gain1 : Gain  Gain=rumori_bias
  Mux : Mux  Inputs=3
  Random Number : RandomNumber  Variance=dev_std_magn_x^2  Seed=7  SampleTime=dt
  Random Number1 : RandomNumber  Variance=dev_std_magn_y^2  Seed=8  SampleTime=dt
  Random Number2 : RandomNumber  Variance=dev_std_magn_z^2  Seed=9  SampleTime=dt
  Scope : Scope  NumInputPorts=3
  Sum : Sum  Inputs=|+++
  bias_magn : Constant  Value=bias_magn
  rotazione campo : MATLAB Function  TreatAsAtomicUnit=on
  m_meas : Outport
  wires:
  rotazione campo/1(m_b) -> Sum/1  "vera"
  R/1 -> rotazione campo/2(R)
  m_I/1 -> rotazione campo/1(m_i)
  Sum/1 -> m_meas/1  "misura"
  Demux/3 -> Scope/3
  Demux/2 -> Scope/2
  bias_magn/1 -> Gain/1  "bias"
  Random Number/1 -> Mux/1  "wn_magn_x"
  Random Number1/1 -> Mux/2  "wn_magn_y"
  Random Number2/1 -> Mux/3  "wn_magn_z"
  Demux/1 -> Scope/1
  Mux/1 -> Gain1/1, Demux/1  "white noise"
  Gain1/1 -> Sum/3
  Gain/1 -> Sum/2

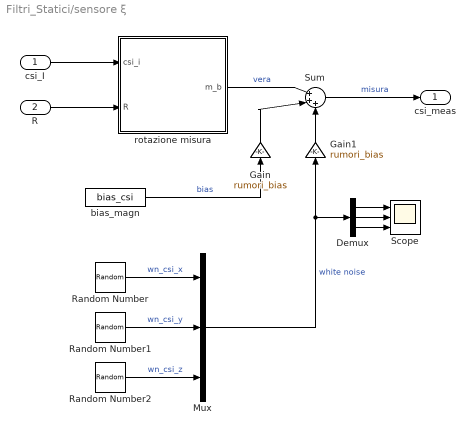
== system Filtri_Statici/sensore ξ  ==
  csi_I : Inport
  R : Inport  Port=2
  Demux : Demux  Outputs=3
  Gain : Gain  Gain=rumori_bias
  Gain1 : Gain  Gain=rumori_bias
  Mux : Mux  Inputs=3
  Random Number : RandomNumber  Variance=dev_std_csi_x^2  Seed=7  SampleTime=dt
  Random Number1 : RandomNumber  Variance=dev_std_csi_y^2  Seed=8  SampleTime=dt
  Random Number2 : RandomNumber  Variance=dev_std_csi_z^2  Seed=9  SampleTime=dt
  Scope : Scope  NumInputPorts=3
  Sum : Sum  Inputs=|+++
  bias_magn : Constant  Value=bias_csi
  rotazione misura : MATLAB Function  TreatAsAtomicUnit=on
  csi_meas : Outport
  wires:
  rotazione misura/1(m_b) -> Sum/1  "vera"
  R/1 -> rotazione misura/2(R)
  csi_I/1 -> rotazione misura/1(csi_i)
  Sum/1 -> csi_meas/1  "misura"
  Demux/3 -> Scope/3
  Demux/2 -> Scope/2
  bias_magn/1 -> Gain/1  "bias"
  Random Number/1 -> Mux/1  "wn_csi_x"
  Random Number1/1 -> Mux/2  "wn_csi_y"
  Random Number2/1 -> Mux/3  "wn_csi_z"
  Demux/1 -> Scope/1
  Mux/1 -> Gain1/1, Demux/1  "white noise"
  Gain1/1 -> Sum/3
  Gain/1 -> Sum/2

== matlab function Filtri_Statici/wrap. ==
  data: u input; y output
function y = wtp(u)

y = wrapToPi(u);

== matlab function Filtri_Statici/wrap, ==
  data: u input; y output
function y = wtp(u)

y = wrapToPi(u);

== matlab function Filtri_Statici/Algoritmo TRIAD ==
  data: m_I input; R_estim output; m_meas input; a_meas input; a_body input; R_esatta input; csi_i input; csi_meas input; check_det_R_estim output; detR_triad output
function [R_estim, check_det_R_estim, detR_triad] = TRIAD(m_I, m_meas, a_meas, a_body, R_esatta,  csi_i, csi_meas)
% Scelgo due vettori non collineari v1 e v2 noti sia in frame body che 
% inerziale su cui basare l'algoritmo
% magnetometro ed accelerometro 
v1_I = m_I;     v1_B = m_meas;  v2_I = R_esatta*a_body;     v2_B = a_meas;
% magnetometro e sensore ξ
% v1_I = m_I;     v1_B = m_meas;  v2_I = csi_i;     v2_B = csi_meas;
% accelerometro e sensore ξ (scelta che porta ad errori minori)
% v1_I = csi_i;     v1_B = csi_meas;  v2_I = R_esatta*a_body;     v2_B = a_meas;

% Definizione delle due triadi
s1 = v1_I;
s2 = cross(v1_I,v2_I)/norm(cross(v1_I,v2_I));
s3 = cross(s1,s2);

r1 = v1_B;
r2 = cross(v1_B,v2_B)/norm(cross(v1_B,v2_B));
r3 = cross(r1,r2);

% Le raccolgo in 2 vettori
% Svect = [s1, s2, s3];
% Rvect = [r1; r2; r3];

% Calcolo la matrice di rotazione
R_estim =s1*r1'+s2*r2'+s3*r3';

det_R_estim = det(R_estim);
if det_R_estim -1 <= 10^-5  % lascio un po di margine per la tolleranzza di calcolo
    check_det_R_estim = 1;
else 
    check_det_R_estim = 0;
end

detR_triad = det(R_estim);

== matlab function Filtri_Statici/cinematica inversa3 ==
  data: R_estim input; phi_estim output; theta_estim output; psi_estim output
function [phi_estim, theta_estim, psi_estim] = inv_kin_estim(R_estim)
% Ricavo gli angoli di Eulero stimati a partire dalla matrice di rotazione
% stimata
phi_estim = atan2(R_estim(3,2),R_estim(3,3));
theta_estim = -atan2(R_estim(3,1),sqrt(R_estim(1,1)^2 + R_estim(2,1)^2));
psi_estim = atan2(R_estim(2,1),R_estim(1,1));

== matlab function Filtri_Statici/Algoritmo Ottimo di Wahba ==
  data: a_meas input; B output; a_body input; R_esatta input; csi_i input; csi_meas input; m_meas input; k_accel parameter; k_csi parameter; k_magn parameter; m_I parameter
function B = WAHBA(a_meas, a_body, R_esatta, csi_i, csi_meas, m_meas, k_accel, k_csi, k_magn, m_I)
% Definisco le grandezze vere poi osservate in terna inerziale
a_I_norm = (R_esatta*a_body)/norm(R_esatta*a_body);     % accelerazione normalizzata veivolo in terna inerziale
csi_I_norm = csi_i/norm(csi_i);                         % misura ξ normalizzata veivolo in terna inerziale 
m_I_norm = m_I/norm(m_I);

% Definisco i vettori delle misure normalizzate
a_meas_norm = a_meas/norm(a_meas);
csi_meas_norm = csi_meas/norm(csi_meas);
m_meas_norm = m_meas/norm(m_meas);

% Si cerca di minimizzare la seguente funzione di costo
%J = 0.5*( k_accel*norm(a_meas-A*a_I)^2 + k_csi*norm(csi_meas-A*csi_I)^2 + k_magn*norm(m_meas-A*m_I) );
% riscrivibile come 
%J = 0.5*( k_accel*(norm(a_I)^2+norm(a_meas)^2)+k_csi*(norm(csi_I)^2+norm(csi_meas)^2)+k_magn*(norm(m_I)^2+norm(m_meas)^2) )- trace(A*B');
% si può allora andare a cercare la A che massimizza la trace(A*B') con 
B = k_accel*a_meas_norm*a_I_norm' + k_csi*csi_meas_norm*csi_I_norm' + k_magn*m_meas_norm*m_I_norm';

== matlab function Filtri_Statici/Soluzione di Farrell, Stuelpnagel & co. ==
  data: B input; R_estim_FS output; check_det output; detR_FS output
function [R_estim_FS, check_det, detR_FS] = Farrell_Stuelpnagel(B)
% Faccio la decomposizione polare della matrice B = U*P
P = (B'*B)^1/2;
U = B/P;
if det(U) > 0
    A_estim = U;
    R_estim_FS = A_estim';
else
    % Decompongo ai valori singolari la matrice simmetrica P
    [W,~,~] = svd(P);
    % Calcolo la matrice ottima A che minimizza il J di Wahba secondo la
    % soluzione di Farrel, Stuelpnagel & co.
    A_estim = U*W*[1, 0, 0;
                   0, 1, 0;
                   0, 0, det(U)]*W';
    R_estim_FS = A_estim';
end

det_R_estim = det(R_estim_FS);
if det_R_estim -1 <= 10^-5  % lascio un po di margine per la tolleranzza di calcolo
    check_det = 1;
else 
    check_det = 0;
end

detR_FS = det(R_estim_FS);

== matlab function Filtri_Statici/cinematica inversa4 ==
  data: R_estim input; phi_estim output; theta_estim output; psi_estim output
function [phi_estim, theta_estim, psi_estim] = inv_kin_estim(R_estim)
% Ricavo gli angoli di Eulero stimati a partire dalla matrice di rotazione
% stimata
phi_estim = atan2(R_estim(3,2),R_estim(3,3));
theta_estim = -atan2(R_estim(3,1),sqrt(R_estim(1,1)^2 + R_estim(2,1)^2));
psi_estim = atan2(R_estim(2,1),R_estim(1,1));

== matlab function Filtri_Statici/Soluzione di Wessner ==
  data: B input; R_estim_W output; detR_W output
function [R_estim_W, detR_W] = Wessner(B)
% Calcolo la soluzione di Wessner al problema di ottimo di Wahba , è un
% caso particolare del problema di Farrell, Stuelpnagel & co.
A_estim = (B')\(B'*B)^1/2; % posso calcorare inv(B) perchè ho 3 vettori misurati non collineari
% A_estim = B*(B'*B)^(0.5);  % formula alternativa equivalente
R_estim_W = A_estim';

% det_R_estim = det(R_estim_W);
% if det_R_estim -1 <= 10^-5  % lascio un po di margine per la tolleranzza di calcolo
%     check_det = 1;
% else 
%     check_det = 0;
% end

detR_W = det(R_estim_W);

== matlab function Filtri_Statici/cinematica inversa5 ==
  data: R_estim input; phi_estim output; theta_estim output; psi_estim output
function [phi_estim, theta_estim, psi_estim] = inv_kin_estim(R_estim)
% Ricavo gli angoli di Eulero stimati a partire dalla matrice di rotazione
% stimata
phi_estim = atan2(R_estim(3,2),R_estim(3,3));
theta_estim = -atan2(R_estim(3,1),sqrt(R_estim(1,1)^2 + R_estim(2,1)^2));
psi_estim = atan2(R_estim(2,1),R_estim(1,1));

== matlab function Filtri_Statici/Soluzione di Davenport ==
  data: B input; R_estim_Dav output; a_meas input; a_body input; R_esatta input; csi_i input; csi_meas input; m_meas input; k_accel parameter; k_csi parameter; k_magn parameter; m_I parameter; flag parameter; index parameter; detR_Dav output
function [R_estim_Dav,detR_Dav] = Davenport(B, a_meas, a_body, R_esatta, csi_i, csi_meas, m_meas, k_accel, k_csi, k_magn, m_I, flag, index)
% Usa i quaternioni per trasformare il problema di Wahba nella ricerca
% dell'autovalore massimo della matrice simmetrica di Davenport K.

% ======================================================================= %
% Definizione delle matrici intermedie per calcolare K
C = B + B';
gamma = trace(B);
    % Definisco i vettori osservati in terna inerziale
a_I = R_esatta*a_body;

z = k_accel*cross(a_meas,a_I) + k_csi*cross(csi_meas,csi_i) + k_magn*cross(m_meas,m_I);

% Definizione della matrice di Davenport
K = [C-gamma*eye(3),    z;
          z',         gamma];   % matrice 4x4 
% ======================================================================= %
% Cerco l'autovalore ed autovettore max della matrice K
[V,D] = eig(K);
[lambda,ind] = sort(diag(D)); %estrae valori sulla diagonale di D e li ordina
    % in ordine crescente nel vettore lambda, ind è il vettore delle permutazioni da fare per ottenere il riordinamento
D_sorted = D(ind,ind);     % riordinamento della matrice D 
V_sorted = V(:,ind);       % riordino V, l'ultima colonna corrisponde allora a quella dell'autovalore massimo
q_max = V_sorted(:,end)/norm(V_sorted(:,end)); % autovettore corrispondente ad autovalore max, corrisponde al quaternione associato ad A_estim
%========== altro metodo non funzionante per trovare q_max ===============%
% lambda = diag(D); 
% 
% % Riordino il vettore degli autovalori dal più grande al più piccolo
% lambda_ord = sort(lambda,'descend','ComparisonMethod','real');
% % for i=1:4 
% %     if imag(lambda_ord(i))<= 10^-6 && flag == 1
% %         index = i;
% %         flag = 0;
% %     end
% % end
% % q_max = V(:,index)/norm(V(:,index)); 
% ======================================================================= %
% Ricavo la matrice di rotazione dal quaternione tramite la formula di
% Rodriguez
    % scompongo il quaternione come q = [s; v] 
s = real(q_max(1));  
v = real(q_max(2:4));
    % non dovrebbero servire i real() perchè sono reali ma vengono definiti
    % in forma complessa con +000000i, real() serve solo per toglierli tale
    % parte immaginaria
S_v = [0,    -v(3), v(2);
       v(3),  0,   -v(1);
      -v(2),  v(1) ,  0];
    % formula di Rodriguez
A_estim = eye(3) + 2*s*S_v + 2*S_v^2; 
% La matrice A così ottenuta in realtà è la trasposta della matrice di
% rotazione che stiamo cercando
R_estim_Dav = A_estim';

% ======================================================================= %
% det_R_estim = det(R_estim_Dav);
% if det_R_estim -1 <= 10^-5  % lascio un po di margine per la tolleranzza di calcolo
%     check_det = 1;
% else 
%     check_det = 0;
% end

detR_Dav = det(R_estim_Dav);

== matlab function Filtri_Statici/cinematica inversa6 ==
  data: R_estim input; phi_estim output; theta_estim output; psi_estim output
function [phi_estim, theta_estim, psi_estim] = inv_kin_estim(R_estim)
% Ricavo gli angoli di Eulero stimati a partire dalla matrice di rotazione
% stimata
phi_estim = atan2(R_estim(3,2),R_estim(3,3));
theta_estim = -atan2(R_estim(3,1),sqrt(R_estim(1,1)^2 + R_estim(2,1)^2));
psi_estim = atan2(R_estim(2,1),R_estim(1,1));

== matlab function Filtri_Statici/wtp ==
  data: u input; y output
function y = wtp(u)

y = wrapToPi(u);

== matlab function Filtri_Statici/Cinematica VTOL, impongo angoli ==
  data: t input; phi output; theta output; psi output; p_dot output; v_dot_i output; a_body output; omega output; R output; g parameter; v_inertial input; e3 parameter; Phi1 parameter; Phi2 parameter; Phi3 parameter; w_phi1 parameter; w_phi2 parameter; w_phi3 parameter; Theta1 parameter; Theta2 parameter; Theta3 parameter; w_theta1 parameter; w_theta2 parameter; w_theta3 parameter; Psi1 parameter; Psi2 parameter; Psi3 parameter; w_psi1 parameter; w_psi2 parameter; w_psi3 parameter; phi_0 parameter; theta_0 parameter; psi_0 parameter
function [phi, theta, psi, p_dot, v_dot_i, a_body, omega, R] = cinematica_esatta_ang(t,g,v_inertial,e3,Phi1, Phi2, Phi3, w_phi1, w_phi2, w_phi3, Theta1, Theta2, Theta3, w_theta1, w_theta2, w_theta3, Psi1, Psi2, Psi3, w_psi1, w_psi2, w_psi3, phi_0, theta_0, psi_0)
% vel_dot è in frame inerziale ed esatta
% v_dot_i è sempre in frame inerziale ma tiene conto dell'errore di
% integrazione numerica di Simulink

% Definizione traiettorie di riferimento
% vel_dot = 10*[-sin(t); -2*sin(2*t); -64*cos(8*t)/128 ]; %traiettoria troppo ricca
vel_dot = zeros(3,1); % approssimazione per VTOL
phi = phi_0+ Phi1*sin(w_phi1*t) + Phi2*sin(w_phi2*t) + Phi3*sin(w_phi3*t);
theta = theta_0+ Theta1*sin(w_theta1*t) + Theta2*sin(w_theta2*t) + Theta3*sin(w_theta3*t);
psi = psi_0 + Psi1*sin(w_psi1*t) + Psi2*sin(w_psi2*t) + Psi3*sin(w_psi3*t);

% Calcolo della velocità angolare a partire dagli angoli di Eulero
dphi = Phi1*w_phi1*cos(w_phi1*t)+Phi2*w_phi2*cos(w_phi2*t)+Phi3*w_phi3*cos(w_phi3*t);
dtheta = Theta1*w_theta1*cos(w_theta1*t)+Theta2*w_theta2*cos(w_theta2*t)+Theta3*w_theta3*cos(w_theta3*t);
dpsi = Psi1*w_psi1*cos(w_psi1*t)+Psi2*w_psi2*cos(w_psi2*t)+Psi3*w_psi3*cos(w_psi3*t);
omega1 = dphi-sin(theta)*dpsi;
omega2 = cos(phi)*dtheta+cos(theta)*sin(phi)*dpsi;
omega3 = -sin(phi)*dtheta+cos(theta)*cos(phi)*dpsi;
omega = [omega1; omega2; omega3];

% Matrice di rotazione da body a inerziale (C_bi in notazione vista a
% lezione) esatta 
R = [cos(theta)*cos(psi),  -cos(phi)*sin(psi) + cos(psi)*sin(phi)*sin(theta),   sin(phi)*sin(psi) + cos(psi)*cos(phi)*sin(theta); 
     cos(theta)*sin(psi),   cos(phi)*cos(psi) + sin(psi)*sin(phi)*sin(theta),  -sin(phi)*cos(psi) + sin(psi)*cos(phi)*sin(theta);
     -sin(theta),           sin(phi)*cos(theta),                                cos(phi)*cos(theta)];
% Definizione accelerazione reale in terna body
a_body = R' * (vel_dot - g*e3); 
% Inverto l'espressione per ricavarne la derivata della velocità in terna inerziale 
v_dot_i =  R*a_body + g*e3;
% Definisco la derivata della posizione come la velocità
p_dot = v_inertial;

== matlab function Filtri_Statici/wtp1 ==
  data: u input; y output
function y = wtp(u)

y = wrapToPi(u);

== matlab function Filtri_Statici/wtp2 ==
  data: u input; y output
function y = wtp(u)

y = wrapToPi(u);

== matlab function Filtri_Statici/wtp3 ==
  data: u input; y output
function y = wtp(u)

y = wrapToPi(u);

== matlab function Filtri_Statici/sensore ξ /rotazione misura ==
  data: csi_i input; m_b output; R input
function m_b = csi_body(csi_i, R)

m_b = R'*csi_i;

== matlab function Filtri_Statici/Cinematica VTOL, impongo omega ==
  data: t input; phi_dot output; phi input; theta input; psi input; theta_dot output; psi_dot output; p_dot output; v_dot_i output; a_body output; omega output; R output; g parameter; v_inertial input; e3 parameter; Omega12 parameter; Omega13 parameter; Omega21 parameter; Omega22 parameter; Omega23 parameter; Omega31 parameter; Omega11 parameter; Omega32 parameter; Omega33 parameter; w_11 parameter; w_12 parameter; w_13 parameter; w_21 parameter; w_22 parameter; w_23 parameter; w_31 parameter; w_32 parameter; w_33 parameter
function [phi_dot, theta_dot, psi_dot, p_dot, v_dot_i, a_body, omega, R] = cinematica_esatta(t, phi,theta,psi, g, v_inertial, e3, Omega12, Omega13, Omega21, Omega22, Omega23, Omega31, Omega11, Omega32, Omega33, w_11, w_12, w_13, w_21, w_22, w_23, w_31, w_32, w_33)
% vel_dot è in frame inerziale ed esatta
% v_dot_i è sempre in frame inerziale ma tiene conto dell'errore di
% integrazione numerica di Simulink

%================ Definizione traiettorie di riferimento =================%
% Moto lineare
% vel_dot = 10*[-sin(t); -2*sin(2*t); -64*cos(8*t)/128 ]; %traiettoria troppo ricca
vel_dot = zeros(3,1); % approssimazione per VTOL
% vel_dot = g/8*[-sin(t); -2*sin(2*t); -64*cos(8*t)/128];  % prova traiettoria lenta

% Moto angolare
omega1 = Omega11*sin(w_11*t) + Omega12*sin(w_12*t) + Omega13*sin(w_13*t);
omega2 = Omega21*sin(w_21*t) + Omega22*sin(w_22*t) + Omega23*sin(w_23*t);
omega3 = Omega31*sin(w_31*t) + Omega32*sin(w_32*t) + Omega33*sin(w_33*t);
omega = [omega1; omega2; omega3];
% omega = zeros(3,1);  % approssimazione per controllare le equazioni

%=================== Cinematica degli angoli di Eulero ===================%
phi_dot = omega(1) + sin(phi)*tan(theta)*omega(2) + cos(phi)*tan(theta)*omega(3);
theta_dot = cos(phi)*omega(2) - sin(phi)*omega(3);
psi_dot = omega(2)*sin(phi)/cos(theta) + omega(3)*cos(phi)/cos(theta);

%=============== Matrice di rotazione da body a inerziale =============== %
% (C_bi in notazione vista a lezione) esatta
R = [cos(theta)*cos(psi),  -cos(phi)*sin(psi) + cos(psi)*sin(phi)*sin(theta),   sin(phi)*sin(psi) + cos(psi)*cos(phi)*sin(theta); 
     cos(theta)*sin(psi),   cos(phi)*cos(psi) + sin(psi)*sin(phi)*sin(theta),  -sin(phi)*cos(psi) + sin(psi)*cos(phi)*sin(theta);
     -sin(theta),           sin(phi)*cos(theta),                                cos(phi)*cos(theta)];

%============== Meccanizzazione delle velocità e posizione ===============%
% Definizione accelerazione reale in terna body
a_body = R' * (vel_dot - g*e3); 
% Inverto l'espressione per ricavarne la derivata della velocità in terna inerziale 
v_dot_i =  R*a_body + g*e3;
% Definisco la derivata della posizione come la velocità
p_dot = v_inertial;

== matlab function Filtri_Statici/magnetometro/rotazione campo ==
  data: m_i input; m_b output; R input
function m_b = magn_body(m_i, R)

m_b = R'*m_i;

== matlab function Filtri_Statici/Metodo QUEST ==
  data: a_meas input; a_body input; R_esatta input; csi_i input; csi_meas input; m_meas input; m_I parameter; k_magn parameter; k_csi parameter; k_accel parameter; B input; R_estim_quest output; check_det_R_estim output
function [R_estim_quest, check_det_R_estim] = QUEST(a_meas, a_body, R_esatta, csi_i, csi_meas, m_meas, m_I, k_magn, k_csi, k_accel, B)
% Risolve numericamente il det(K-lambda*I_4) = 0 o equivalentemente 
% risolvere lamda^4 - (a+b)*lamda^2 -c*lambda + (a*b+c*gamma-d) = 0
% Definizione delle matrici intermedie
C = B + B';
gamma = trace(B);
    % Definisco i vettori osservati in terna inerziale
    a_I = R_esatta*a_body;
    
z = k_accel*cross(a_meas,a_I) + k_csi*cross(csi_meas,csi_i) + k_magn*cross(m_meas,m_I);

% Dichiaro adjoint() come una funzione estrinseca, serve per farla funzionare
% coder.extrinsic('adjoint')
% C_adj = adjoint(C); 
C_adj = det(C)*eye(size(C))/(C);  % metodo alternativo per trovare l'aggiunta di una matrice

a = gamma^2 - trace(C_adj);
b = gamma^2 + norm(z)^2;
c = det(C) + z'*C*z;
d = z'*(C^2)*z;

lambda_0 = k_accel + k_csi + k_magn;

% Definizione della funzione da risolvere
fun = @(lambda) lambda^4 - (a+b)*lambda^2 -c*lambda + (a*b+c*gamma-d); 
% Risolvo
lambda_max = fzero(fun,lambda_0);

% Ridefinisco la matrice di Davenport per trovare l'autovettore associato a
% lambda_max
K = [C-gamma*eye(3),    z;
          z',         gamma];   % matrice 4x4 
% Trova l'autovettore corrispondente all'autovalore noto
[V, D] = eig(K);
index = find(diag(D) == lambda_max);
q_max = V(:, index);

% Ricavo la matrice di rotazione dal quaternione tramite la formula di
% Rodriguez
    % scompongo il quaternione come q = [s; v] 
s = real(q_max(1));  
v = real(q_max(2:4));
% non dovrebbero servire i real() perchè dovrebbero essere già reali ma così non è,
% che sia causato dalla presenza dei rumori sulle misure? No, anche senza
% restano complessi
S_v = [0,    -v(3), v(2);
       v(3),  0,   -v(1);
      -v(2),  v(1) ,  0];
    % formula di Rodriguez
A_estim = eye(3) + 2*s*S_v + 2*S_v^2; 
% La matrice A così ottenuta in realtà è la trasposta della matrice di
% rotazione che stiamo cercando
R_estim_quest = A_estim';

det_R_estim_quest = det(R_estim_quest);
if det_R_estim_quest -1 <= 10^-5  % lascio un po di margine per la tolleranzza di calcolo
    check_det_R_estim = 1;
else 
    check_det_R_estim = 0;
end

== matlab function Filtri_Statici/cinematica inversa1 ==
  data: R_estim input; phi_estim output; theta_estim output; psi_estim output
function [phi_estim, theta_estim, psi_estim] = inv_kin_estim(R_estim)
% Ricavo gli angoli di Eulero stimati a partire dalla matrice di rotazione
% stimata
phi_estim = atan2(R_estim(3,2),R_estim(3,3));
theta_estim = -atan2(R_estim(3,1),sqrt(R_estim(1,1)^2 + R_estim(2,1)^2));
psi_estim = atan2(R_estim(2,1),R_estim(1,1));

== matlab function Filtri_Statici/wrapToPi ==
  data: u input; y output
function y = wtp(u)

y = wrapToPi(u);

== matlab function Filtri_Statici/, ==
  data: u input; y output
function y = wtp(u)

y = wrapToPi(u);

== matlab function Filtri_Statici/wrap ==
  data: u input; y output
function y = wtp(u)

y = wrapToPi(u);
